simulink model "Xe_chay_theo_quy_dao_R"  (R2021b)
settings: Solver=VariableStepAuto  StartTime=0.0  StopTime=30  RelTol=1e-3
libraries: simulink_extras x1
settings Model: Creator=HL_1810  LastModifiedBy=ASUS

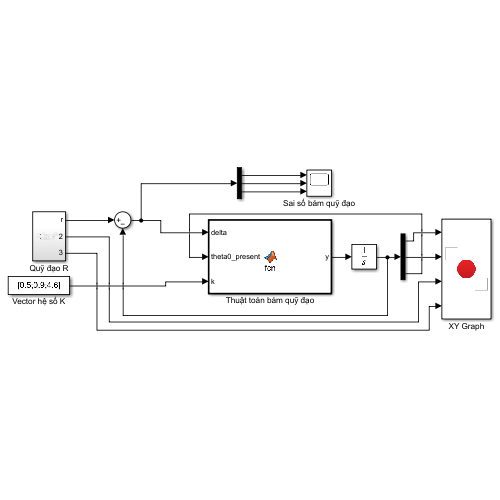
[thumbnail: Simulink's stored preview of the top-level diagram]
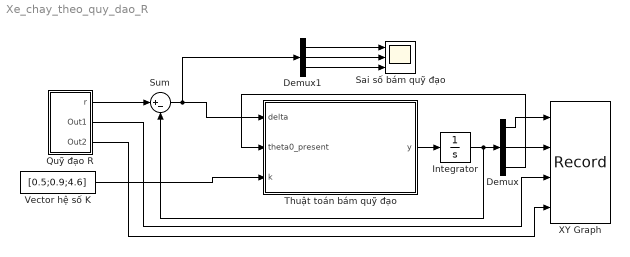
== system Xe_chay_theo_quy_dao_R ==
  Demux : Demux  Outputs=3
  Demux1 : Demux  Outputs=3
  Integrator : Integrator  InitialCondition=[2.18;1;pi/2]
  Quỹ đạo R : Subsystem
  Sai số bám quỹ đạo : Scope  NumInputPorts=3
  Sum : Sum  Inputs=|+-
  Thuật toán bám quỹ đạo : MATLAB Function  TreatAsAtomicUnit=on
  Vector hệ số K : Constant  Value=[0.5;0.9;4.6]  VectorParams1D=off
  XY Graph : Record  FileSettingsInternal="{\"entries\":[{\"content\":{\"excelSettings\":{\"content\":{},\"type\":\"Streamout.ExcelSettings\"}},\"type\":\"Streamout.FileSettingStorage\",\"uuid\":\"6114f7b0-9e14-440a-81fa-28d0fd3fbdce\"}],\"packageUris\":[\"http://schema.mathworks.com/mf0/streamout_blocks/R2020a\"],\"version\":\"1.0\"}"  Layout=[1 1]  SignalsInternal="{\"entries\":[{\"content\":{\"signals\":[{\"content\":{\"blockPath\":[\"Xe_chay_theo_quy_dao_R/XY Graph\"],\"channel\":[],\"dimensions\":[1],\"domain\":\"Xe_chay_theo_quy_dao_R/XY Graph\",\"lineColor\":\"#edb120\",\"plots\":[1],\"port\":1,\"sid\":[\"\"],\"signalID\":4597,\"signalName\":\"Quy dao Robot\"},\"type\":\"RecordBlkView.Signal\",\"uuid\":\"0892df32-1b73-4b5b-b7ee-86954f94a307\"},{\"content\":{\"blockPath\":[\"Xe_chay_theo_quy_dao_R/XY Graph\"],\"channel\":[],\"dimensions\":[1],\"domain\":\"Xe_chay_theo_quy_dao_R/XY Graph\",\"lineColor\":\"#7e2f8e\",\"plots\":[1],\"port\":2,\"sid\":[\"\"],\"signalID\":4601,\"signalName\":\"Quy dao Robot\"},\"type\":\"RecordBlkView.Signal\",\"uuid\":\"e3fd8502-4d2d-47bd-9f0a-e6bd6108e795\"},{\"content\":{\"blockPath\":[\"Xe_chay_theo_quy_dao_R/XY Graph\"],\"channel\":[],\"dimensions\":[1],\"domain\":\"Xe_chay_theo_quy_dao_R/XY Graph\",\"lineColor\":\"#77ac30\",\"plots\":[1,2],\"port\":3,\"sid\":[\"\"],\"signalID\":4605,\"signalName\":\"Quỹ đạo R:2\"},\"type\":\"RecordBlkView.Signal\",\"uuid\":\"762e54f1-c4ab-4d5e-861e-41f4a4bcc7c3\"},{\"content\":{\"blockPath\":[\"Xe_chay_theo_quy_dao_R/XY Graph\"],\"channel\":[],\"dimensions\":[1],\"domain\":\"Xe_chay_theo_quy_dao_R/XY Graph\",\"lineColor\":\"#4dbeee\",\"plots\":[1,2],\"port\":4,\"sid\":[\"\"],\"signalID\":4609,\"signalName\":\"Quỹ đạo R:3\"},\"type\":\"RecordBlkView.Signal\",\"uuid\":\"7ecca508-7e54-4c33-a2d3-0b14d8672526\"}]},\"type\":\"RecordBlkView.InputSignals\",\"uuid\":\"3b93ac5a-0b8f-4397-ba43-f6877f5b2789\"}],\"packageUris\":[\"http://schema.mathworks.com/mf0/streamout_blocks/R2020a\"],\"version\":\"1.0\"}"  VisualizationBindings="{\"xyplotplugin\":{\"info\":[{\"series\":[{\"bindingParametersList\":[{\"parameter\":\"X-Axis\",\"signalID\":4597,\"signalName\":\"Quy dao Robot\"},{\"parameter\":\"Y-Axis\",\"signalID\":4601,\"signalName\":\"Quy dao Robot\"}],\"seriesID\":14118},{\"bindingParametersList\":[{\"parameter\":\"Y-Axis\",\"signalID\":4609,\"signalName\":\"Quá»¹ Ä‘áº¡o R:3\"},{\"parameter\":\"X-Axis\",\"signalID\":4605,\"signalName\":\"Quá»¹ Ä‘áº¡o R:2\"}],\"seriesID\":27318}],\"subplotID\":1},{\"series\":[{\"bindingParametersList\":[{\"parameter\":\"X-Axis\",\"signalID\":4605,\"signalName\":\"Quá»¹ Ä‘áº¡o R:2\"},{\"parameter\":\"Y-Axis\",\"signalID\":4609,\"signalName\":\"Quá»¹ Ä‘áº¡o R:3\"}],\"seriesID\":33639}],\"subplotID\":2}]}}"  CompatibilityTag=XY
  wires:
  Demux/2 -> XY Graph/2
  Quỹ đạo R/3(Out2) -> XY Graph/4
  Demux/1 -> XY Graph/1
  Demux/3 -> Thuật toán bám quỹ đạo/2(theta0_present)
  Integrator/1 -> Sum/2, Demux/1
  Thuật toán bám quỹ đạo/1(y) -> Integrator/1
  Sum/1 -> Demux1/1, Thuật toán bám quỹ đạo/1(delta)
  Quỹ đạo R/1(r) -> Sum/1
  Quỹ đạo R/2(Out1) -> XY Graph/3
  Vector hệ số K/1 -> Thuật toán bám quỹ đạo/3(k)
  Demux1/1 -> Sai số bám quỹ đạo/1
  Demux1/2 -> Sai số bám quỹ đạo/2
  Demux1/3 -> Sai số bám quỹ đạo/3

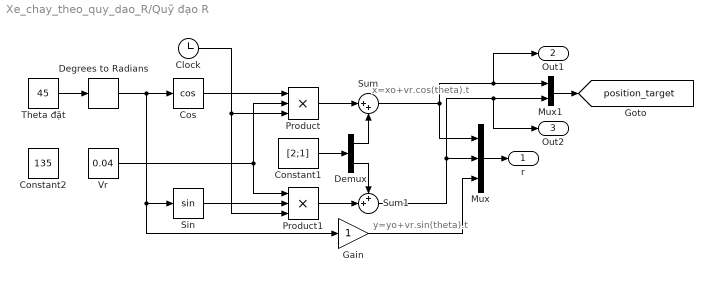
== system Xe_chay_theo_quy_dao_R/Quỹ đạo R ==
  note: y=yo+vr.sin(theta).t
  note: x=xo+vr.cos(theta).t
  Clock : Clock
  Constant1 : Constant  Value=[2;1]
  Constant2 : Constant  Value=135
  Cos : Trigonometry  Operator=cos
  Degrees to Radians : simulink_extras/Transformations/Degrees to Radians
  Demux : Demux  Outputs=2
  Gain : Gain
  Mux : Mux  Inputs=3
  Mux1 : Mux  Inputs=2
  Product : Product  Inputs=3
  Product1 : Product  Inputs=3
  Sin : Trigonometry
  Sum : Sum  Inputs=|++
  Sum1 : Sum  Inputs=++|
  Theta đặt : Constant  Value=45
  Vr : Constant  Value=0.04
  r : Outport
  Out1 : Outport  Port=2
  Out2 : Outport  Port=3
  tag scope: position_target=global
  wires:
  Sum1/1 -> Mux/2, Out2/1, Mux1/2
  Constant1/1 -> Demux/1
  Theta đặt/1 -> Degrees to Radians/1
  Clock/1 -> Product1/3, Product/3
  Cos/1 -> Product/1
  Degrees to Radians/1 -> Sin/1, Gain/1, Cos/1
  Sin/1 -> Product1/2
  Sum/1 -> Out1/1, Mux1/1, Mux/1
  Gain/1 -> Mux/3
  Product1/1 -> Sum1/2
  Vr/1 -> Product/2, Product1/1
  Product/1 -> Sum/1
  Demux/2 -> Sum1/1
  Demux/1 -> Sum/2
  Mux/1 -> r/1
  Mux1/1 -> [position_target]

== matlab function Xe_chay_theo_quy_dao_R/Thuật toán bám quỹ đạo ==
  data: delta input; y output; theta0_present input; k input
function y= fcn(delta,theta0_present,k)
%#codegen
A=[cos(theta0_present)   sin(theta0_present) 0;
    -sin(theta0_present) cos(theta0_present) 0;
    0                    0                    1];
e=A*delta;
V_c=[0.04*cos(e(3))+k(1)*e(1);
    0+k(2)*0.04*e(2)+k(3)*0.04*sin(e(3))];

Matrix=[cos(theta0_present) 0;
        sin(theta0_present) 0;
        0                   1];
u=Matrix*V_c;
y = u;
